simulink model "zustandsRegler"  (R2019b)
settings: Solver=VariableStepAuto  StartTime=0.0  StopTime=20  MaxStep=1e-3  RelTol=1e-3
values from neighbouring files (symbols this model uses):
  A = [a11, a12, a13, a14, a15; a21, a22, a23, a24, a25; a31, a32, a33, a34,     a35; a41, a42, a43, a44, a45; a51, a52, a53, a54, a55]    [initial_data.m]
  B = [b11; b12; b13; b14; b15]    [initial_data.m]
  C = [c11, c12, c13, c14, c15]    [initial_data.m]
  K = lqr(system, Q, R)    [initial_data.m]

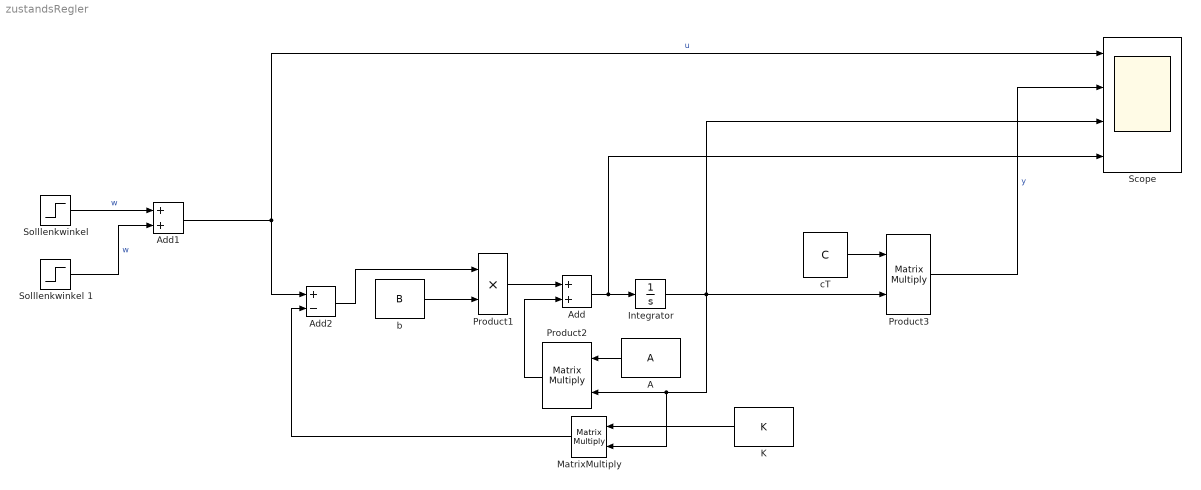
== system zustandsRegler ==
  A : Constant  Value=A  VectorParams1D=off
  Add : Sum
  Add1 : Sum
  Add2 : Sum  Inputs=+-
  Integrator : Integrator
  K : Constant  Value=K  VectorParams1D=off
  MatrixMultiply : Product  Multiplication=Matrix(*)
  Product1 : Product
  Product2 : Product  Multiplication=Matrix(*)
  Product3 : Product  Multiplication=Matrix(*)
  Scope : Scope  NumInputPorts=4
  "Solllenkwinkel " : Step  Time=5  SampleTime=0
  Solllenkwinkel 1 : Step  Time=10  After=-1  SampleTime=0
  b : Constant  Value=B  VectorParams1D=off
  cT : Constant  Value=C  VectorParams1D=off
  wires:
  Add/1 -> Scope/4, Integrator/1
  Product1/1 -> Add/1
  Product2/1 -> Add/2
  b/1 -> Product1/2
  A/1 -> Product2/1
  Integrator/1 -> Product3/2, Scope/3, Product2/2, MatrixMultiply/2
  cT/1 -> Product3/1
  Add1/1 -> Scope/1, Add2/1  "u"
  "Solllenkwinkel "/1 -> Add1/1  "w"
  Solllenkwinkel 1/1 -> Add1/2  "w"
  Product3/1 -> Scope/2  "y"
  Add2/1 -> Product1/1
  MatrixMultiply/1 -> Add2/2
  K/1 -> MatrixMultiply/1
